simulink model "week3_prob3"  (R2020a)
settings: Solver=ode15s  StartTime=0.0  StopTime=10  RelTol=1e-3
PreLoadFcn:
  | ms = 300.5;
  | MU = 40.3;
  | ks = 17474.9;
  | kt = 179913;
  | cs = 1328;
  | ct = 3.70;
undefined symbols (not defined in the file): sigbuilder_block
settings Model: Creator=akhil singh  LastModifiedBy=akhil singh

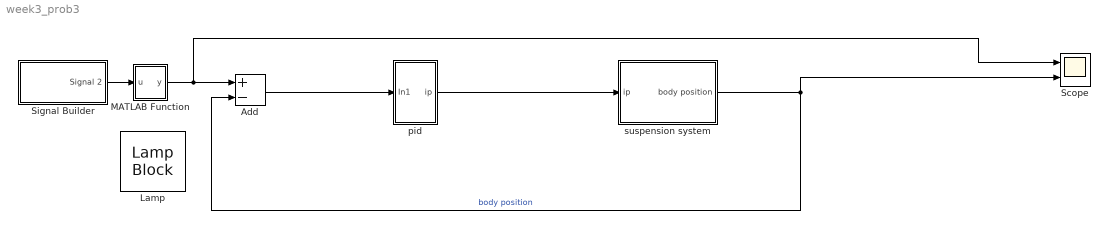
== system week3_prob3 ==
  Add : Sum  Inputs=+-
  Lamp : LampBlock
  MATLAB Function : MATLAB Function  TreatAsAtomicUnit=on
  Scope : Scope  NumInputPorts=2
  Signal Builder : Subsystem  Tag=STV Subsys  LoadFcn=sigbuilder_block('load');  StartFcn=sigbuilder_block('start');  StopFcn=sigbuilder_block('stop');  ClipboardFcn=sigbuilder_block('clipboard');  mask(Sigbuilder block){tuvar=[0:10]}
      mask help: Simulink:masks:SigbuilderBlock_MD
      mask init:
      | if ~strcmp(get_param(bdroot(gcbh),'SimulationStatus'),'stopped') tuvar = sigbuilder_block('maskInit'); end
      settings: CopyFcn=sigbuilder_block('copy');  DeleteFcn=sigbuilder_block('delete');  ModelCloseFcn=sigbuilder_block('modelClose');  PreSaveFcn=sigbuilder_block('preSave');  PauseFcn=sigbuilder_block('pause');  ContinueFcn=sigbuilder_block('continue');  NameChangeFcn=sigbuilder_block('namechange');  OpenFcn=sigbuilder_block('open',[267 153 721 359.25 ]);  CloseFcn=sigbuilder_block('close');
      mask Display: plot(0, 0, 100, 100,[2, 2, 32, 32, 2], [68, 8, 8, 68, 68],[32, 2], [38, 38], [32, 19, 2],[53, 60, 44], [32, 17, 17, 2],[16, 16, 31, 31]);txt = getActiveGroup(gcbh);text(2, 100, txt,'verticalAlignment', 'top');
  pid : Subsystem
  suspension system : Subsystem
  wires:
  Signal Builder/1(Signal 2) -> MATLAB Function/1(u)
  suspension system/1(body position) -> Scope/2, Add/2  "body position"
  Add/1 -> pid/1(In1)
  pid/1(ip) -> suspension system/1(ip)
  MATLAB Function/1(y) -> Scope/1, Add/1

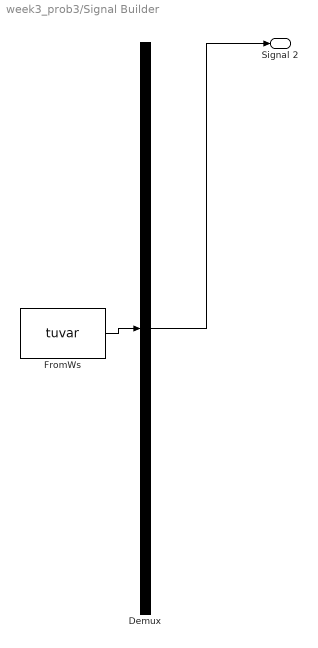
== system week3_prob3/Signal Builder ==
  Demux : Demux  Tag=STV Demux  Outputs=1
      settings: DisplayOption=none
  FromWs : FromWorkspace  Tag=STV FromWs  VariableName=tuvar
      SigBuilderData=|
      | common.afterFinalStr = 'Extrapolate'
      | common.sampleTime = 0
      | dataSet.timeRange = [0 10]
      | dataSet.name = 'Group 1'
      | sbobj.Groups.Name = 'Group 1'
      | sbobj.Groups.Signals.Name = 'Signal 2'
      | sbobj.Groups.Signals.XData = [0 1 1 2 2 3.52 3.52 4 4 5.52 5.52 6 6 7 7 8 8 9 9 10]
      | sbobj.Groups.Signals.YData = [0.94 0.94 0 1.02 2 1.02 0 0 2 -0.02 -2.02 -2.02 2 2 -2 0 2 2 0.96 0]
  Signal 2 : Outport  Tag=STV Outport
  wires:
  FromWs/1 -> Demux/1
  Demux/1 -> Signal 2/1

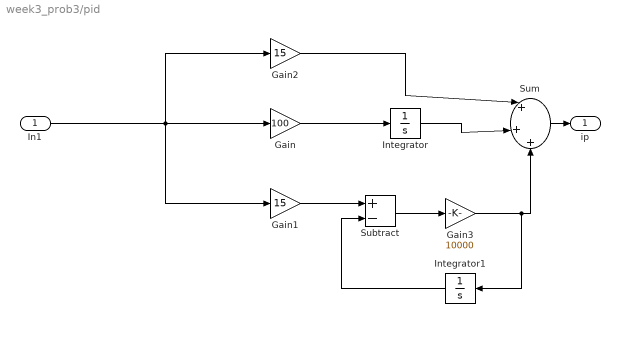
== system week3_prob3/pid ==
  In1 : Inport
  Gain : Gain  Gain=100
  Gain1 : Gain  Gain=15
  Gain2 : Gain  Gain=15
  Gain3 : Gain  Gain=10000
  Integrator : Integrator
  Integrator1 : Integrator
  Subtract : Sum  Inputs=+-
  Sum : Sum  Inputs=|+|+|+
  ip : Outport
  wires:
  Sum/1 -> ip/1
  Gain/1 -> Integrator/1
  Gain2/1 -> Sum/1
  Gain1/1 -> Subtract/1
  Integrator/1 -> Sum/2
  In1/1 -> Gain1/1, Gain/1, Gain2/1
  Integrator1/1 -> Subtract/2
  Gain3/1 -> Integrator1/1, Sum/3
  Subtract/1 -> Gain3/1

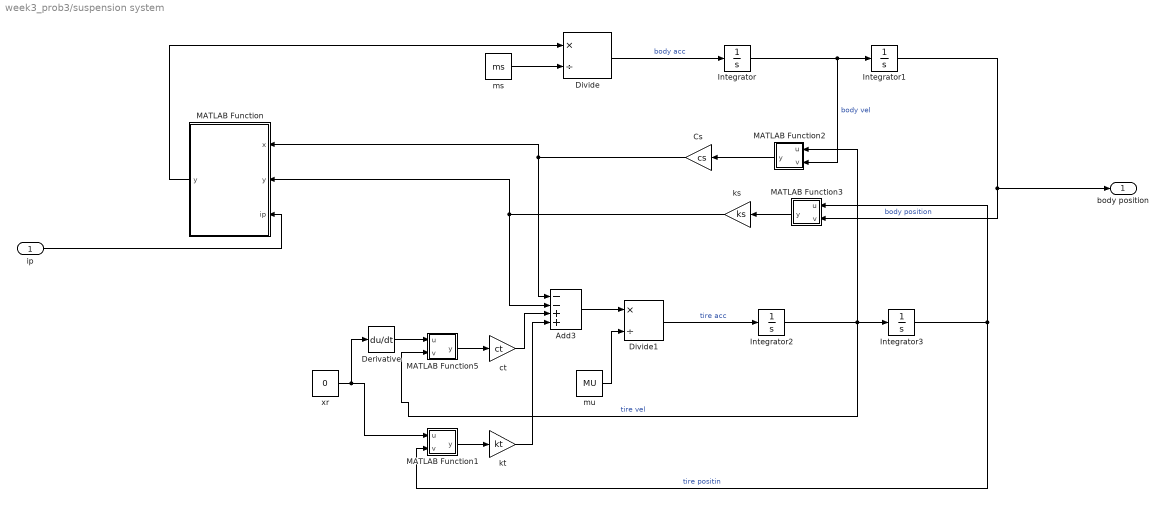
== system week3_prob3/suspension system ==
  ip : Inport
  Add3 : Sum  Inputs=--++
  Cs : Gain  Gain=cs
  Derivative : Derivative
  Divide : Product  Inputs=*/
  Divide1 : Product  Inputs=*/
  Integrator{,1..3} (4 alike) : Integrator
  MATLAB Function : MATLAB Function  TreatAsAtomicUnit=on
  MATLAB Function1 : MATLAB Function  TreatAsAtomicUnit=on
  MATLAB Function2 : MATLAB Function  TreatAsAtomicUnit=on
  MATLAB Function3 : MATLAB Function  TreatAsAtomicUnit=on
  MATLAB Function5 : MATLAB Function  TreatAsAtomicUnit=on
  ct : Gain  Gain=ct
  ks : Gain  Gain=ks
  kt : Gain  Gain=kt
  ms : Constant  Value=ms
  mu : Constant  Value=MU
  xr : Constant  Value=0
  body position : Outport
  wires:
  xr/1 -> MATLAB Function1/1(u), Derivative/1
  Integrator2/1 -> MATLAB Function2/1(u), MATLAB Function5/2(v), Integrator3/1  "tire vel"
  ms/1 -> Divide/2
  Integrator/1 -> MATLAB Function2/2(v), Integrator1/1  "body vel"
  Integrator1/1 -> body position/1, MATLAB Function3/2(v)  "body position"
  Integrator3/1 -> MATLAB Function1/2(v), MATLAB Function3/1(u)  "tire positin"
  mu/1 -> Divide1/2
  ct/1 -> Add3/3
  MATLAB Function/1(y) -> Divide/1
  Cs/1 -> MATLAB Function/1(x), Add3/1
  ks/1 -> MATLAB Function/2("y "), Add3/2
  Add3/1 -> Divide1/1
  kt/1 -> Add3/4
  Divide1/1 -> Integrator2/1  "tire acc"
  Divide/1 -> Integrator/1  "body acc"
  Derivative/1 -> MATLAB Function5/1(u)
  MATLAB Function5/1(y) -> ct/1
  MATLAB Function3/1(y) -> ks/1
  MATLAB Function2/1(y) -> Cs/1
  MATLAB Function1/1(y) -> kt/1
  ip/1 -> MATLAB Function/3(ip)

== matlab function week3_prob3/suspension system/MATLAB Function ==
  data: x input; y output; y input; ip input
function y = fcn(x, y, ip)

y = x+y+ip;

== matlab function week3_prob3/suspension system/MATLAB Function2 ==
  data: u input; y output; v input
function y = fcn(u, v)

y = u-v;

== matlab function week3_prob3/suspension system/MATLAB Function3 ==
  data: u input; y output; v input
function y = fcn(u, v)

y = u-v;

== matlab function week3_prob3/MATLAB Function ==
  data: u input; y output
function y = fcn(u)

if u > 0
    y = 1;
elseif u < 0    
    y = -1;
else
    y = 0;
end

== matlab function week3_prob3/suspension system/MATLAB Function5 ==
  data: u input; y output; v input
function y = fcn(u, v)

y = u-v;

== matlab function week3_prob3/suspension system/MATLAB Function1 ==
  data: u input; y output; v input
function y = fcn(u, v)

y = u-v;
